simulink model "fault model"  (R2019a)
settings: Solver=VariableStepAuto  StartTime=0.0  StopTime=0.5  RelTol=1e-3
libraries: powerlib x16
settings Model: Creator=Arun Nair  LastModifiedBy=Arun Nair

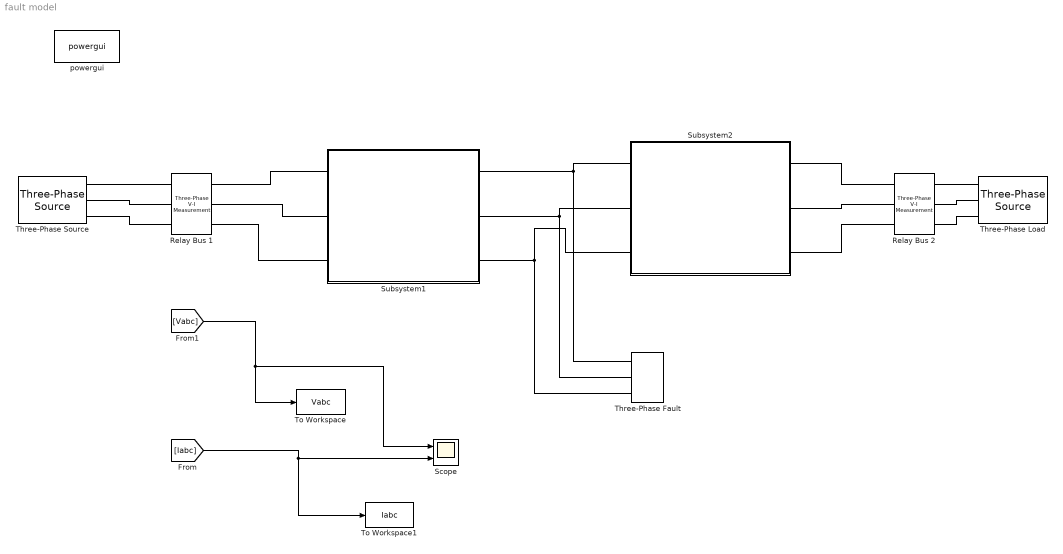
== system fault model ==
  "Relay Bus 1 " : powerlib/Measurements/Three-Phase V-I Measurement  VoltageMeasurement=phase-to-phase  SetLabelV=on  LabelV=Vabc  Vpu=on  VpuLL=off  CurrentMeasurement=yes  SetLabelI=on  LabelI=Iabc  Ipu=on  Pbase=100e6  Vbase=500e3  OutputType=Complex  PhasorSimulation=off  PSBequivalent=0
      settings: SourceProductName=Simscape Electrical
  "Relay Bus 2 " : powerlib/Measurements/Three-Phase V-I Measurement  VoltageMeasurement=no  SetLabelV=on  LabelV=Vabc  Vpu=on  VpuLL=off  CurrentMeasurement=no  SetLabelI=on  LabelI=Iabc  Ipu=on  Pbase=100e6  Vbase=500e3  OutputType=Complex  PhasorSimulation=off  PSBequivalent=0
      settings: SourceProductName=Simscape Electrical
  "Scope " : Scope  NumInputPorts=2
  "Subsystem1 " : Subsystem
  "Subsystem2 " : Subsystem
  "Three-Phase Fault " : powerlib/Elements/Three-Phase Fault  InitialStates=0  FaultA=on  FaultB=on  FaultC=on  GroundFault=off  SwitchTimes="[1/50  5/50]"  External=off  SwitchStatus=NaN  FaultResistance=0.001  GroundResistance=0.01  SnubberResistance=1e6  SnubberCapacitance=inf  Measurements=None
      settings: SourceProductName=Simscape Electrical
  "Three-Phase Load " : powerlib/Electrical Sources/Three-Phase Source  InternalConnection=Yg  VoltagePhases=on  Voltage=500e3  PhaseAngle=-30  Voltage_phases=[25e3 25e3 25e3]/sqrt(3)  PhaseAngles_phases=[0 -120 +120]  Frequency=50  NonIdealSource=on  SpecifyImpedance=on  Resistance=0.8929  Inductance=16.58e-3  ShortCircuitLevel=100e6  BaseVoltage=500e3  XRratio=7  BusType=swing  Pref=10e3  Qref=0  Prefabc=[10e3, 10e3, 10e3]  Qrefabc=[0, 0, 0]  Qmin=-inf  Qmax=inf
      settings: SourceProductName=Simscape Electrical
  "Three-Phase Source " : powerlib/Electrical Sources/Three-Phase Source  InternalConnection=Yg  VoltagePhases=on  Voltage=500e3  PhaseAngle=0  Voltage_phases=[25e3 25e3 25e3]/sqrt(3)  PhaseAngles_phases=[0 -120 +120]  Frequency=50  NonIdealSource=on  SpecifyImpedance=off  Resistance=0.8929  Inductance=16.58e-3  ShortCircuitLevel=100e6  BaseVoltage=500e3  XRratio=7  BusType=swing  Pref=10e3  Qref=0  Prefabc=[10e3, 10e3, 10e3]  Qrefabc=[0, 0, 0]  Qmin=-inf  Qmax=inf
      settings: SourceProductName=Simscape Electrical
  "To Workspace " : ToWorkspace  VariableName=Vabc  SaveFormat=Timeseries
  "To Workspace1 " : ToWorkspace  VariableName=Iabc  SaveFormat=Timeseries
  powergui : powerlib/powergui  Priority=1  SimulationMode=Discrete  SampleTime=3e-5  frequency=60  Iterations=50  frequencyindice=50  Pbase=100e6  ErrMax=1e-4  UnitsV=kV  UnitsW=MW  buscounter=0  FunctionMessages=off  echomessages=off  EnableUseOfTLC=off  CurrentSourceSwitches=off  DisableSnubberDevices=off  DisableRonSwitches=off  DisableVfSwitches=off  DisplayEquations=off  AutomaticDiscreteSolvers=off  SolverType=Tustin/Backward Euler (TBE)  Interpol=off  ExternalGateDelay=off  methode=off  Ts=100  x0status=blocks  SPID=on  SwTol=0  HookPort=off  NonlinearTolerance=0  nMaxIteration=15  ContinueOnMaxIteration=off  RestoreLinks=warning  ResistiveCurrentMeasurement=off  Frange=[0:2:500]  Ylog=off  Xlog=on  ShowGrid=off  save=off  variable=ZData  structure=0  ZoomFFT=off  StartTime=0.0  cycles=1  DisplayStyle=1  fundamental=60  FreqAxis=off  MaxFrequency=1000  frequencyindicesteady=1  RmsSteady=1  display=off
      settings: SourceProductName=Simscape Electrical
  wires:
  [Iabc] -> "Scope "/2, "To Workspace1 "/1
  [Vabc] -> "To Workspace "/1, "Scope "/1
  connections:
  "Subsystem2 "/RConn1 -- "Three-Phase Fault "/LConn1 -- "Subsystem1 "/RConn1
  "Subsystem2 "/RConn3 -- "Three-Phase Fault "/LConn3 -- "Subsystem1 "/RConn3
  "Subsystem2 "/RConn2 -- "Three-Phase Fault "/LConn2 -- "Subsystem1 "/RConn2
  "Relay Bus 1 "/RConn1 -- "Subsystem1 "/LConn1
  "Relay Bus 1 "/LConn1 -- "Three-Phase Source "/RConn1
  "Relay Bus 1 "/RConn3 -- "Subsystem1 "/LConn3
  "Subsystem2 "/LConn1 -- "Relay Bus 2 "/LConn1
  "Subsystem2 "/LConn3 -- "Relay Bus 2 "/LConn3
  "Subsystem2 "/LConn2 -- "Relay Bus 2 "/LConn2
  "Three-Phase Source "/RConn3 -- "Relay Bus 1 "/LConn3
  "Three-Phase Source "/RConn2 -- "Relay Bus 1 "/LConn2
  "Relay Bus 1 "/RConn2 -- "Subsystem1 "/LConn2
  "Relay Bus 2 "/RConn1 -- "Three-Phase Load "/RConn1
  "Relay Bus 2 "/RConn2 -- "Three-Phase Load "/RConn2
  "Relay Bus 2 "/RConn3 -- "Three-Phase Load "/RConn3

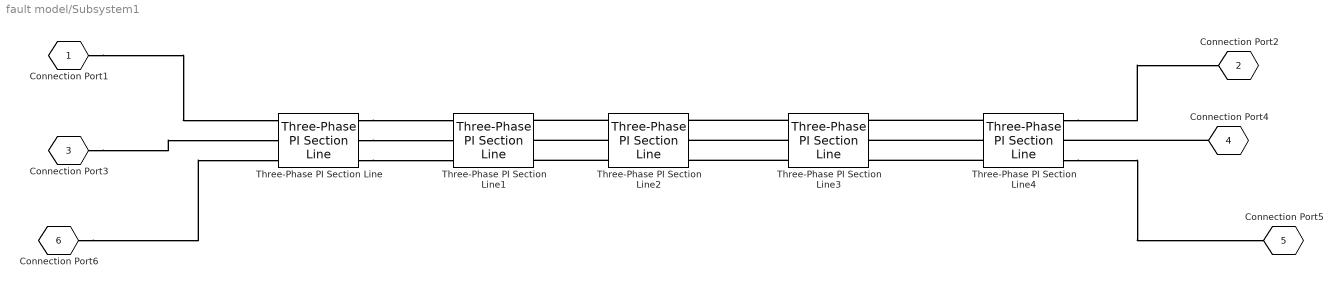
== system fault model/Subsystem1  ==
  Three-Phase PI Section Line{,1..4} (5 alike) : powerlib/Elements/Three-Phase PI Section Line  LConnTagsString=a|b|c  RConnTagsString=A|B|C  Frequency=50  Resistances=[ 0.01273 0.3864]  Inductances="[ 0.9337e-3  4.1264e-3]"  Capacitances=[12.74e-9 7.751e-9]  Length=30
      settings: SourceProductName=Simscape Electrical
  "Connection Port1 " : PMIOPort  Tag=PMCPort  Side=Left
  "Connection Port2 " : PMIOPort  Tag=PMCPort  Port=2  Side=Right
  "Connection Port3 " : PMIOPort  Tag=PMCPort  Port=3  Side=Left
  "Connection Port4 " : PMIOPort  Tag=PMCPort  Port=4  Side=Right
  "Connection Port5 " : PMIOPort  Tag=PMCPort  Port=5  Side=Right
  "Connection Port6 " : PMIOPort  Tag=PMCPort  Port=6  Side=Left
  connections:
  "Connection Port6 "/RConn1 -- Three-Phase PI Section Line/LConn3
  Three-Phase PI Section Line4/LConn3 -- Three-Phase PI Section Line3/RConn3
  Three-Phase PI Section Line2/LConn3 -- Three-Phase PI Section Line1/RConn3
  Three-Phase PI Section Line4/LConn1 -- Three-Phase PI Section Line3/RConn1
  Three-Phase PI Section Line/RConn1 -- Three-Phase PI Section Line1/LConn1
  Three-Phase PI Section Line4/LConn2 -- Three-Phase PI Section Line3/RConn2
  Three-Phase PI Section Line4/RConn1 -- "Connection Port2 "/RConn1
  Three-Phase PI Section Line/RConn3 -- Three-Phase PI Section Line1/LConn3
  Three-Phase PI Section Line2/LConn2 -- Three-Phase PI Section Line1/RConn2
  Three-Phase PI Section Line4/RConn3 -- "Connection Port5 "/RConn1
  Three-Phase PI Section Line2/LConn1 -- Three-Phase PI Section Line1/RConn1
  Three-Phase PI Section Line3/LConn2 -- Three-Phase PI Section Line2/RConn2
  Three-Phase PI Section Line3/LConn1 -- Three-Phase PI Section Line2/RConn1
  Three-Phase PI Section Line3/LConn3 -- Three-Phase PI Section Line2/RConn3
  "Connection Port1 "/RConn1 -- Three-Phase PI Section Line/LConn1
  "Connection Port3 "/RConn1 -- Three-Phase PI Section Line/LConn2
  "Connection Port4 "/RConn1 -- Three-Phase PI Section Line4/RConn2
  Three-Phase PI Section Line/RConn2 -- Three-Phase PI Section Line1/LConn2

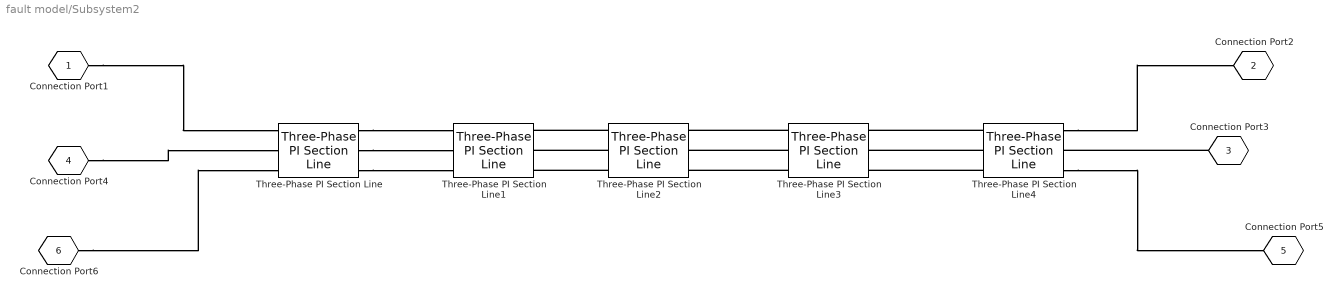
== system fault model/Subsystem2  ==
  Three-Phase PI Section Line{,1..4} (5 alike) : powerlib/Elements/Three-Phase PI Section Line  LConnTagsString=a|b|c  RConnTagsString=A|B|C  Frequency=50  Resistances=[ 0.01273 0.3864]  Inductances="[ 0.9337e-3  4.1264e-3]"  Capacitances=[12.74e-9 7.751e-9]  Length=30
      settings: SourceProductName=Simscape Electrical
  "Connection Port1 " : PMIOPort  Tag=PMCPort  Side=Left
  "Connection Port2 " : PMIOPort  Tag=PMCPort  Port=2  Side=Right
  "Connection Port3 " : PMIOPort  Tag=PMCPort  Port=3  Side=Right
  "Connection Port4 " : PMIOPort  Tag=PMCPort  Port=4  Side=Left
  "Connection Port5 " : PMIOPort  Tag=PMCPort  Port=5  Side=Right
  "Connection Port6 " : PMIOPort  Tag=PMCPort  Port=6  Side=Left
  connections:
  Three-Phase PI Section Line/RConn2 -- Three-Phase PI Section Line1/LConn2
  "Connection Port3 "/RConn1 -- Three-Phase PI Section Line4/RConn2
  "Connection Port4 "/RConn1 -- Three-Phase PI Section Line/LConn2
  "Connection Port1 "/RConn1 -- Three-Phase PI Section Line/LConn1
  Three-Phase PI Section Line3/LConn3 -- Three-Phase PI Section Line2/RConn3
  Three-Phase PI Section Line3/LConn1 -- Three-Phase PI Section Line2/RConn1
  Three-Phase PI Section Line3/LConn2 -- Three-Phase PI Section Line2/RConn2
  Three-Phase PI Section Line2/LConn1 -- Three-Phase PI Section Line1/RConn1
  Three-Phase PI Section Line4/RConn3 -- "Connection Port5 "/RConn1
  Three-Phase PI Section Line2/LConn2 -- Three-Phase PI Section Line1/RConn2
  Three-Phase PI Section Line/RConn3 -- Three-Phase PI Section Line1/LConn3
  Three-Phase PI Section Line4/RConn1 -- "Connection Port2 "/RConn1
  Three-Phase PI Section Line4/LConn2 -- Three-Phase PI Section Line3/RConn2
  Three-Phase PI Section Line/RConn1 -- Three-Phase PI Section Line1/LConn1
  Three-Phase PI Section Line4/LConn1 -- Three-Phase PI Section Line3/RConn1
  Three-Phase PI Section Line2/LConn3 -- Three-Phase PI Section Line1/RConn3
  Three-Phase PI Section Line4/LConn3 -- Three-Phase PI Section Line3/RConn3
  "Connection Port6 "/RConn1 -- Three-Phase PI Section Line/LConn3
